simulink model "Lab_model_laplace"  (R2025b)
settings: Solver=VariableStepAuto  StartTime=0.0  StopTime=t_stop  RelTol=1e-3
undefined symbols (not defined in the file): c1, c2, c3, k1, k2, k3, m1, m2, m3
settings Model: Creator=LEGION  LastModifiedBy=LEGION
settings DataIOCC: ReturnWorkspaceOutputs=off

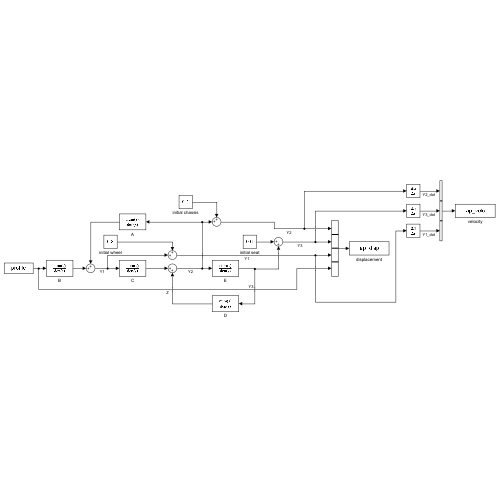
[thumbnail: Simulink's stored preview of the top-level diagram]
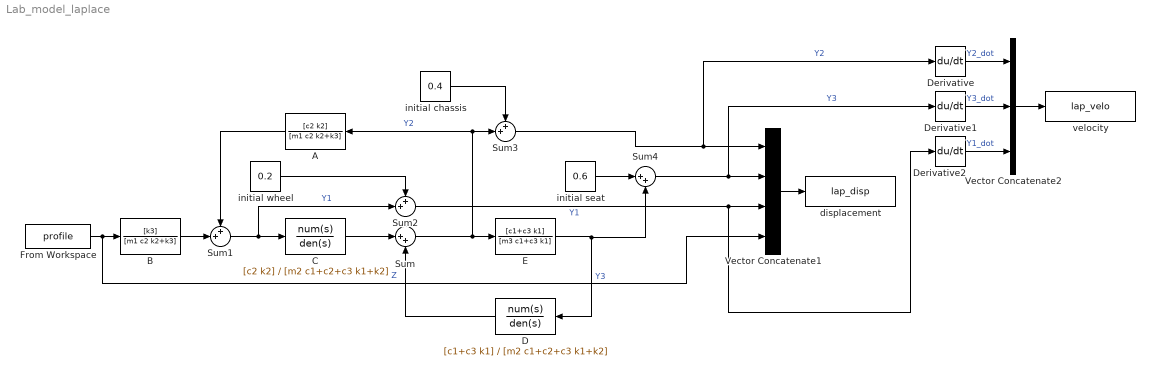
== system Lab_model_laplace ==
  A : TransferFcn  Numerator=[c2 k2]  Denominator=[m1 c2 k2+k3]
  B : TransferFcn  Numerator=[k3]  Denominator=[m1 c2 k2+k3]
  C : TransferFcn  Numerator=[c2 k2]  Denominator=[m2 c1+c2+c3 k1+k2]
  D : TransferFcn  Numerator=[c1+c3 k1]  Denominator=[m2 c1+c2+c3 k1+k2]
  Derivative : Derivative
  Derivative1 : Derivative
  Derivative2 : Derivative
  E : TransferFcn  Numerator=[c1+c3 k1]  Denominator=[m3 c1+c3 k1]
  From Workspace : FromWorkspace  VariableName=profile
  Sum : Sum  Inputs=|++
  Sum1 : Sum  Inputs=++|
  Sum2 : Sum  Inputs=++|
  Sum3 : Sum  Inputs=++|
  Sum4 : Sum  Inputs=|++
  Vector Concatenate1 : Concatenate  NumInputs=4
  Vector Concatenate2 : Concatenate  NumInputs=3
  displacement : ToWorkspace  VariableName=lap_disp  SaveFormat=Structure With Time  SampleTime=-1
  initial chassis : Constant  Value=0.4
  initial seat : Constant  Value=0.6
  initial wheel : Constant  Value=0.2
  velocity : ToWorkspace  VariableName=lap_velo  SaveFormat=Structure With Time  SampleTime=-1
  wires:
  E/1 -> Sum4/2, D/1  "Y3"
  D/1 -> Sum/2
  C/1 -> Sum/1
  Sum1/1 -> Sum2/2, C/1  "Y1"
  Sum/1 -> A/1, Sum3/2, E/1  "Y2"
  A/1 -> Sum1/1
  B/1 -> Sum1/2
  From Workspace/1 -> Vector Concatenate1/4, B/1  "Z"
  initial chassis/1 -> Sum3/1
  Sum3/1 -> Vector Concatenate1/1, Derivative/1  "Y2"
  Sum4/1 -> Vector Concatenate1/2, Derivative1/1  "Y3"
  initial seat/1 -> Sum4/1
  Sum2/1 -> Vector Concatenate1/3, Derivative2/1  "Y1"
  initial wheel/1 -> Sum2/1
  Vector Concatenate1/1 -> displacement/1
  Derivative1/1 -> Vector Concatenate2/2  "Y3_dot"
  Derivative2/1 -> Vector Concatenate2/3  "Y1_dot"
  Derivative/1 -> Vector Concatenate2/1  "Y2_dot"
  Vector Concatenate2/1 -> velocity/1
